simulink model "tn2"  (R2018a)
settings: Solver=FixedStepAuto  StartTime=0.0  StopTime=100.0  FixedStep=0.005  RelTol=1e-3
values from neighbouring files (symbols this model uses):
  b = m2*l1*l2    (= 0.001665)    [pend_model_init.m]
undefined symbols (not defined in the file or in its folder): A, F0, J, K, Kd, Ki, Kp, lm, lp, M, phi0
libraries: simulink x1
settings Model: Creator=DELL  LastModifiedBy=DELL

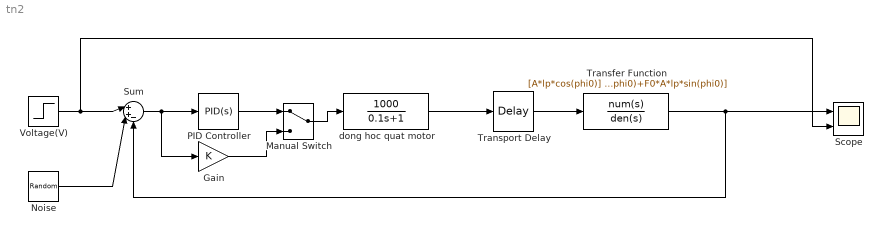
== system tn2 ==
  Gain : Gain  Gain=K
  Manual Switch : ManualSwitch
  "Noise " : RandomNumber  Variance=0.001  SampleTime=0.1
  PID Controller : simulink/Continuous/PID Controller  Controller=PID  TimeDomain=Continuous-time  SampleTime=-1  IntegratorMethod=Forward Euler  FilterMethod=Forward Euler  Form=Parallel  UseFilter=on  ControllerParametersSource=internal  P=Kp  I=Ki  D=Kd  N=100  InitialConditionSource=internal  InitialConditionForIntegrator=0  InitialConditionForFilter=0  ExternalReset=none  LimitOutput=off  UpperSaturationLimit=inf  LowerSaturationLimit=-inf  LinearizeAsGain=on  AntiWindupMode=none  Kb=1  TrackingMode=off  Kt=1  PParamMin=[]  PParamMax=[]  IParamMin=[]  IParamMax=[]  DParamMin=[]  DParamMax=[]  NParamMin=[]  NParamMax=[]  KbParamMin=[]  KbParamMax=[]  KtParamMin=[]  KtParamMax=[]  POutMin=[]  POutMax=[]  IOutMin=[]  IOutMax=[]  DOutMin=[]  DOutMax=[]  NOutMin=[]  NOutMax=[]  KbOutMin=[]  KbOutMax=[]  KtOutMin=[]  KtOutMax=[]  IntegratorOutMin=[]  IntegratorOutMax=[]  FilterOutMin=[]  FilterOutMax=[]  SumOutMin=[]  SumOutMax=[]  SumI1OutMin=[]  SumI1OutMax=[]  SumI2OutMin=[]  SumI2OutMax=[]  SumI3OutMin=[]  SumI3OutMax=[]  SumDOutMin=[]  SumDOutMax=[]  SaturationOutMin=[]  SaturationOutMax=[]  IntegratorContinuousStateAttributes=''  IntegratorStateMustResolveToSignalObject=off  IntegratorRTWStateStorageClass=Auto  FilterContinuousStateAttributes=''  FilterStateMustResolveToSignalObject=off  FilterRTWStateStorageClass=Auto  DifferentiatorICPrevScaledInput=0  DifferentiatorOutMin=[]  DifferentiatorOutMax=[]  FilterDiffOutCoefMin=[]  FilterDiffOutCoefMax=[]  SumDenOutMin=[]  SumDenOutMax=[]  SumNumOutMin=[]  SumNumOutMax=[]  ReciprocalOutMin=[]  ReciprocalOutMax=[]  DivideOutMin=[]  DivideOutMax=[]  TunerSelectOption=Transfer Function Based (PID Tuner App)
  Scope : Scope  NumInputPorts=2
  Sum : Sum  Inputs=|++-
  Transfer Function : TransferFcn  Numerator=[A*lp*cos(phi0)]  Denominator=[J b M*9.81*lm*cos(phi0)+F0*A*lp*sin(phi0)]
  Transport Delay : TransportDelay  DelayTime=0.02
  Voltage(V) : Step  After=5  SampleTime=0
  dong hoc quat motor : TransferFcn  Numerator=1000  Denominator=[0.1 1]
  wires:
  Transport Delay/1 -> Transfer Function/1
  dong hoc quat motor/1 -> Transport Delay/1
  "Noise "/1 -> Sum/2
  Voltage(V)/1 -> Scope/2, Sum/1
  PID Controller/1 -> Manual Switch/1
  Manual Switch/1 -> dong hoc quat motor/1
  Sum/1 -> Gain/1, PID Controller/1
  Gain/1 -> Manual Switch/2
  Transfer Function/1 -> Scope/1, Sum/3
